simulink model "DatosIdent"  (R2023b)
settings: Solver=VariableStepAuto  StartTime=0.0  StopTime=10.0  RelTol=1e-3
libraries: SignalEditorBlockLib x1
settings Model: Creator=Hajar  LastModifiedBy=Hajar
settings DebuggingCC: ParameterPrecisionLossMsg=none

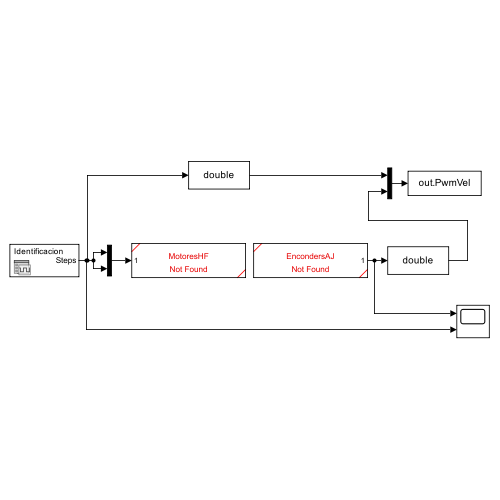
[thumbnail: Simulink's stored preview of the top-level diagram]
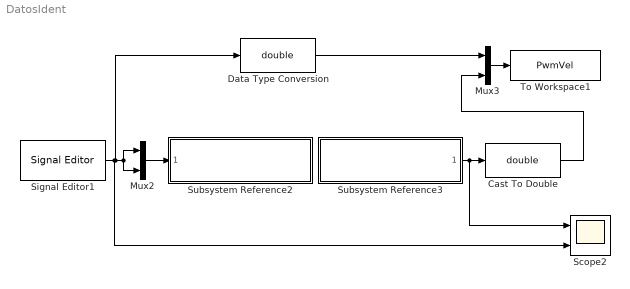
== system DatosIdent ==
  Cast To Double : DataTypeConversion  OutDataTypeStr=double  SaturateOnIntegerOverflow=off  RndMeth=Floor
  Data Type Conversion : DataTypeConversion  OutDataTypeStr=double  SaturateOnIntegerOverflow=off  RndMeth=Floor
  Mux2 : Mux  Inputs=2
  Mux3 : Mux  Inputs=2
  Scope2 : Scope  NumInputPorts=2
  Signal Editor1 : SignalEditorBlockLib/Signal Editor  FileName=C:\€RA2024\HFpiero\AntiguData\Rampa.mat  ActiveScenario=Identificacion  ActiveSignal=Steps  IsBus=off  OutputBusObjectStr=Bus: BusObject  SampleTime=0  ZeroCross=off  OutputAfterFinalValue=Setting to zero  Unit=inherit  PreserveSignalName=on  ApplySigPropsToAllScenarios=on  ApplySigPropsToAllSignals=off
  Subsystem Reference2 : Subsystem  ReferencedSubsystem=MotoresHF
  Subsystem Reference3 : Subsystem  ReferencedSubsystem=EncondersAJ
  To Workspace1 : ToWorkspace  VariableName=PwmVel  SampleTime=-1
      settings: Save2DSignal=2-D array (concatenate along first dimension)
  wires:
  Mux2/1 -> Subsystem Reference2/1
  Mux3/1 -> To Workspace1/1
  Cast To Double/1 -> Mux3/2
  Data Type Conversion/1 -> Mux3/1
  Subsystem Reference3/1 -> Scope2/1, Cast To Double/1
  Signal Editor1/1 -> Scope2/2, Data Type Conversion/1, Mux2/1, Mux2/2
